simulink model "Rakete"  (Simulink 7.7)
settings: Solver=ode45  StartTime=0.0  StopTime=10.0  RelTol=1e-3
undefined symbols (not defined in the file): Durchsatz_1, Durchsatz_2, m1_leer, m2_leer, SchubProDurchsatz, St1_Treibstoff, St2_Treibstoff
settings Model: Creator=karo  LastModifiedBy=hexren
settings DebuggingCC: FcnCallInpInsideContextMsg=Enable All
settings GRTTargetCC: CombineOutputUpdateFcns=on

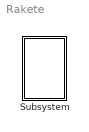
== system Rakete ==
  Subsystem : Subsystem

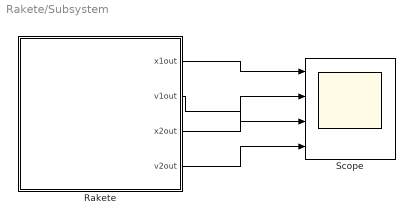
== system Rakete/Subsystem ==
  Rakete : Stateflow chart  TreatAsAtomicUnit=on
  Scope : Scope  NumInputPorts=4
      settings: YMin=-5~-5~-5~-5  YMax=5~5~5~5
  wires:
  Rakete/1(x1out) -> Scope/1
  Rakete/3(x2out) -> Scope/2
  Rakete/2(v1out) -> Scope/3
  Rakete/4(v2out) -> Scope/4

== stateflow chart Subsystem/Rakete ==
  state StufenGemeinsam
    du:
    // Derivatives
    [v1_dor v2_dot] = Acc1();
    x1_dot = v1;
    x2_dot = v2;
    m1_dot = -Durchsatz_1;
    m2_dot = 0;
    // Output
    x1_out = x1;
    v1_out = v1;
    x2_out = x2;
    v2_out = v2;
  state Ende
  (default) -> StufenGemeinsam : {Init();}
  StufenGemeinsam -> Ende : [m1 <= m1_leer]
      | {m1 = m1_leer}
  data: a1 function_output double; a2 function_output double; m1_leer parameter double; m2_leer parameter double; St1_Treibstoff parameter double; St2_Treibstoff parameter double; Durchsatz_1 parameter double; Durchsatz_2 parameter double; SchubProDurchsatz parameter double; x1 local double; x2 local double; v1 local double; v2 local double; m1 local double; m2 local double; x1out output double; v1out output double; x2out output double; v2out output double; Erdmasse constant double =5.9736*10^24; Erdradius constant double =6378000; Gravitationskonstante constant double =66.743*10^-12
  data x1 settings: updateMethod=SF_CONTINUOUS_TIME_DATA
  data x2 settings: updateMethod=SF_CONTINUOUS_TIME_DATA
  data v1 settings: updateMethod=SF_CONTINUOUS_TIME_DATA
  data v2 settings: updateMethod=SF_CONTINUOUS_TIME_DATA
  data m1 settings: updateMethod=SF_CONTINUOUS_TIME_DATA
  data m2 settings: updateMethod=SF_CONTINUOUS_TIME_DATA
  function Init:
    | function Init
    |     x1 = 0;
    |     x2 = 0;
    |     v1 = 0;
    |     v2 = 0;
    |     m1 = m1_leer + St1_Treibstoff;
    |     m2 = m2_leer + St2_Treibstoff;
    | end
  function [a1,a2] = Acc1:
    | function [a1,a2] = Acc1
    |     Schubkraft = Durchsatz_1 * SchubProDurchsatz;
    |     mRakete = m1 + m2;
    |     entfernung = Erdradius + x1;
    |     FS = Gravitationskonstante * ((Erdmasse + mRakete) / (entfernung^2));
    |     
    |     a1 = (Schubkraft - FS)/ mRakete;
    |     a2 = a1;
    | end
